simulink library "eventcameralib"  (R2023a)
settings: Solver=VariableStepAuto  StartTime=0.0  StopTime=10.0  RelTol=1e-3
settings Model: Creator=csaunder  LastModifiedBy=csaunder
settings ModelReferenceCC: UpdateModelReferenceTargets=IfOutOfDate
settings RTWCC: GPUComputeCapability=5.0
settings ConfigComp: CovBoundaryAbsTol=1.0e-5

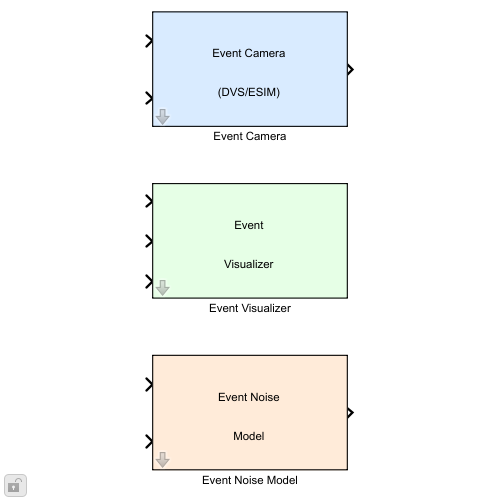
[thumbnail: Simulink's stored preview of the top-level diagram]
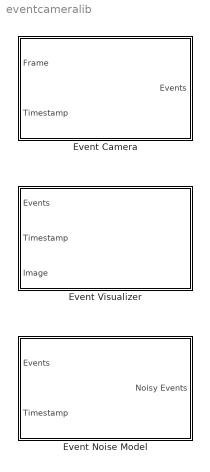
== system eventcameralib ==
  Event Camera : Subsystem  mask(Event Camera){ContrastThresholdOn=0.2, ContrastThresholdOff=0.2, MaxEventsPerFrame=500000, RefractoryPeriod=0, BandwidthHz=Inf, ThresholdMismatch=0, PixelLatency=100e-6}
      mask prompts: ContrastThresholdOn "ON threshold (C+)"; ContrastThresholdOff "OFF threshold (C-)"; MaxEventsPerFrame "Max events per frame"; RefractoryPeriod "Refractory period (s)"; BandwidthHz "Pixel bandwidth (Hz)"; ThresholdMismatch "Threshold mismatch (std dev)"; PixelLatency "Latency (s)"
      mask help: DVS event camera simulator. Converts intensity frames to asynchronous events [x, y, timestamp, polarity].
      mask Help: DVS event camera simulator. Converts grayscale or RGB intensity frames to asynchronous events [x, y, timestamp, polarity] by detecting threshold crossings in log-intensity space.
      mask DialogControl MainTab Prompt: Main
      mask DialogControl ContrastThresholdOn Tooltip: Log-intensity increase that triggers an ON (+1) event. Typical range: 0.1-0.5.
      mask DialogControl ContrastThresholdOff Tooltip: Log-intensity decrease that triggers an OFF (-1) event. Typical range: 0.1-0.5.
      mask DialogControl MaxEventsPerFrame Tooltip: Upper bound on total events per frame to prevent runaway output. Increase for high-resolution sensors.
      mask DialogControl AdvancedTab Prompt: Advanced
      mask DialogControl RefractoryPeriod Tooltip: Per-pixel dead time (seconds) after firing before the pixel can fire again. Set to 0 to disable.
      mask DialogControl BandwidthHz Tooltip: First-order low-pass cutoff (Hz) on log-intensity per pixel. Models limited analog bandwidth. Set to Inf to disable.
      mask DialogControl ThresholdMismatch Tooltip: Standard deviation of per-pixel Gaussian variation on thresholds. Models fixed-pattern noise. Set to 0 to disable.
      mask Display:
      | port_label('input', 1, 'Frame');
      | port_label('input', 2, 'Time');
      | port_label('output', 1, 'Events');
      | color('black');
      | patch([0.1 0.9 0.9 0.1], [0.1 0.1 0.9 0.9], [0.85 0.92 1.0]);
      | text(0.5, 0.62, 'Event Camera', 'horizontalAlignment', 'center');
      | text(0.5, 0.35, '(DVS/ESIM)', 'horizontalAlignment', 'center');
  Event Noise Model : Subsystem  mask(Event Noise Model){ImageHeight=240, ImageWidth=320, BackgroundRate=0, TimestampJitter=0, NumHotPixels=0, HotPixelRate=1000, LeakRate=0, MaxEventsPerStep=500000}
      mask prompts: ImageHeight "Image height (pixels)"; ImageWidth "Image width (pixels)"; BackgroundRate "Background noise (events/s)"; TimestampJitter "Timestamp jitter std dev (s)"; NumHotPixels "Number of hot pixels"; HotPixelRate "Hot pixel rate (events/s/pixel)"; LeakRate "Leak rate (events/s/pixel)"; MaxEventsPerStep "Max events per step"
      mask help: Post-processing noise model for DVS event streams.
      mask Help: Post-processing noise model for DVS event streams. Adds background noise, hot pixels, timestamp jitter, and leak-rate drift to ideal event output.
      mask DialogControl MainTab Prompt: Main
      mask DialogControl ImageHeight Tooltip: Sensor height in pixels. Must match the input event coordinate range.
      mask DialogControl ImageWidth Tooltip: Sensor width in pixels. Must match the input event coordinate range.
      mask DialogControl BackgroundRate Tooltip: Rate of random spurious events across the entire sensor (events/s). Set to 0 to disable.
      mask DialogControl TimestampJitter Tooltip: Standard deviation of Gaussian noise added to event timestamps (seconds). Set to 0 to disable.
      mask DialogControl AdvancedTab Prompt: Advanced
      mask DialogControl NumHotPixels Tooltip: Number of fixed pixels that fire constantly regardless of scene content. Set to 0 to disable.
      mask DialogControl HotPixelRate Tooltip: Firing rate of each hot pixel (events/s/pixel).
      mask DialogControl LeakRate Tooltip: Slow reference drift rate causing spurious events in static regions (events/s/pixel). Set to 0 to disable.
      mask DialogControl MaxEventsPerStep Tooltip: Upper bound on total output events per time step including injected noise.
      mask Display:
      | port_label('input', 1, 'Events');
      | port_label('input', 2, 'Time');
      | port_label('output', 1, 'Noisy Events');
      | color('black');
      | patch([0.1 0.9 0.9 0.1], [0.1 0.1 0.9 0.9], [1.0 0.92 0.85]);
      | text(0.5, 0.62, 'Event Noise', 'horizontalAlignment', 'center');
      | text(0.5, 0.35, 'Model', 'horizontalAlignment', 'center');
  Event Visualizer : Subsystem  mask(Event Visualizer){ImageHeight=240, ImageWidth=320, TimeSurfaceDecay=0.3}
      mask prompts: ImageHeight "Image height (pixels)"; ImageWidth "Image width (pixels)"; TimeSurfaceDecay "Time surface decay (s)"
      mask help: Real-time 3-panel event camera visualization (raw camera, polarity frame, time surface).
      mask Help: Real-time 3-panel visualization: raw camera image, polarity frame (blue=ON, red=OFF), and exponential-decay time surface.
      mask DialogControl SettingsTab Prompt: Settings
      mask DialogControl ImageHeight Tooltip: Sensor height in pixels. Must match the camera resolution.
      mask DialogControl ImageWidth Tooltip: Sensor width in pixels. Must match the camera resolution.
      mask DialogControl TimeSurfaceDecay Tooltip: Exponential decay time constant (seconds) for the time surface display. Smaller values fade faster.
      mask Display:
      | port_label('input', 1, 'Events');
      | port_label('input', 2, 'Time');
      | port_label('input', 3, 'Image');
      | color('black');
      | patch([0.1 0.9 0.9 0.1], [0.1 0.1 0.9 0.9], [0.9 1.0 0.9]);
      | text(0.5, 0.62, 'Event', 'horizontalAlignment', 'center');
      | text(0.5, 0.35, 'Visualizer', 'horizontalAlignment', 'center');

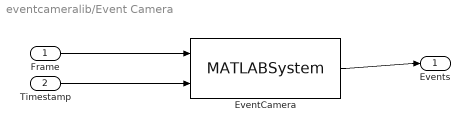
== system eventcameralib/Event Camera ==
  Frame : Inport
  Timestamp : Inport  Port=2
  EventCamera : MATLABSystem  System=EventCamera  ContrastThresholdOn=ContrastThresholdOn  ContrastThresholdOff=ContrastThresholdOff  RefractoryPeriod=RefractoryPeriod  ThresholdMismatch=ThresholdMismatch  BandwidthHz=BandwidthHz  Latency=PixelLatency  LogEpsilon=1e-3  MaxEventsPerFrame=MaxEventsPerFrame  SimulateUsing=Interpreted execution
      mask Type: EventCamera
      mask Display:
      | disp('EventCamera');
      | port_label('input',1,'frame');
      | port_label('input',2,'timestamp');
      | port_label('output',1,'events');
  Events : Outport
  wires:
  Frame/1 -> EventCamera/1
  Timestamp/1 -> EventCamera/2
  EventCamera/1 -> Events/1

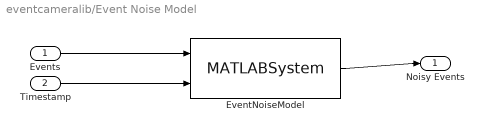
== system eventcameralib/Event Noise Model ==
  Events : Inport
  Timestamp : Inport  Port=2
  EventNoiseModel : MATLABSystem  System=EventNoiseModel  ImageHeight=ImageHeight  ImageWidth=ImageWidth  BackgroundRate=BackgroundRate  NumHotPixels=NumHotPixels  HotPixelRate=HotPixelRate  TimestampJitter=TimestampJitter  LeakRate=LeakRate  MaxEventsPerStep=MaxEventsPerStep  SimulateUsing=Interpreted execution
      mask Type: EventNoiseModel
      mask Display:
      | disp('EventNoiseModel');
      | port_label('input',1,'events');
      | port_label('input',2,'timestamp');
      | port_label('output',1,'noisyEvents');
  Noisy Events : Outport
  wires:
  Events/1 -> EventNoiseModel/1
  Timestamp/1 -> EventNoiseModel/2
  EventNoiseModel/1 -> Noisy Events/1

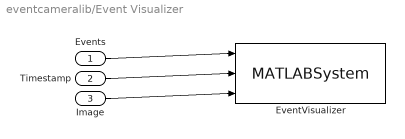
== system eventcameralib/Event Visualizer ==
  Events : Inport
  Timestamp : Inport  Port=2
  Image : Inport  Port=3
  EventVisualizer : MATLABSystem  System=EventVisualizer  ImageHeight=ImageHeight  ImageWidth=ImageWidth  TimeSurfaceDecay=TimeSurfaceDecay  SimulateUsing=Interpreted execution
      mask Type: EventVisualizer
      mask Display:
      | disp('EventVisualizer');
      | port_label('input',1,'events');
      | port_label('input',2,'timestamp');
      | port_label('input',3,'cameraImage');
  wires:
  Events/1 -> EventVisualizer/1
  Timestamp/1 -> EventVisualizer/2
  Image/1 -> EventVisualizer/3
